simulink model "PID_discreto_vs_continuo(1)"  (R2022b)
settings: Solver=VariableStepAuto  StartTime=0.0  StopTime=5  RelTol=1e-3
undefined symbols (not defined in the file or in its folder): DiscIntNeverNeededParam
libraries: cstblocks x2, simulink x1
settings Model: Creator=57317  LastModifiedBy=Duván Ramírez Lotta

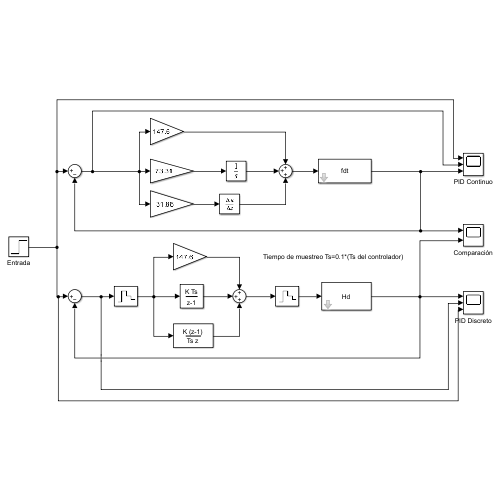
[thumbnail: Simulink's stored preview of the top-level diagram]
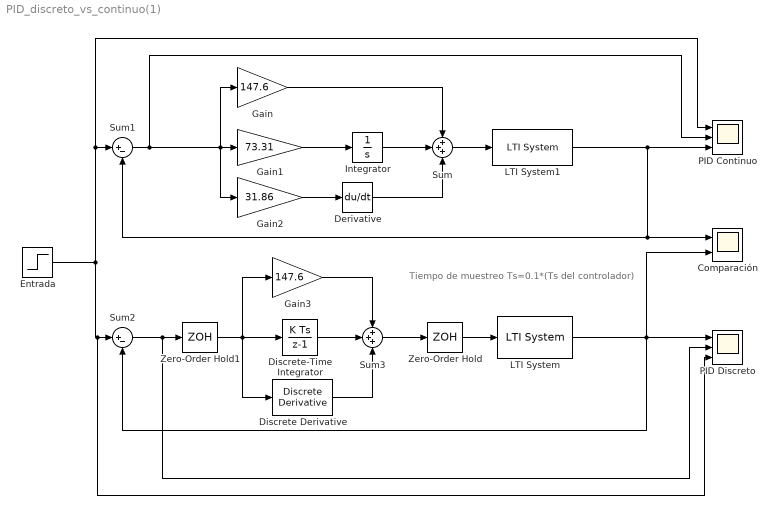
== system PID_discreto_vs_continuo(1) ==
  note: Tiempo de muestreo Ts=0.1*(Ts del controlador)
  Comparación : Scope  NumInputPorts=2
  Derivative : Derivative
  Discrete Derivative : simulink/Discrete/Discrete Derivative  gainval=31.86  ICPrevScaledInput=0.0  OutMin=[]  OutMax=[]  OutDataType=fixdt(1, 16)  OutScaling=2^-10  DoSatur=off
  Discrete-Time Integrator : DiscreteIntegrator  gainval=73.31  SampleTime=0.0001  ICPrevOutput=DiscIntNeverNeededParam  ICPrevScaledInput=DiscIntNeverNeededParam
  Entrada : Step  SampleTime=0
  Gain : Gain  Gain=147.6
  Gain1 : Gain  Gain=73.31
  Gain2 : Gain  Gain=31.86
  Gain3 : Gain  Gain=147.6
  Integrator : Integrator
  LTI System : cstblocks/LTI System  sys=Hd  IC=[]
  LTI System1 : cstblocks/LTI System  sys=fdt  IC=[]
  PID Continuo : Scope  NumInputPorts=3
  PID Discreto : Scope  NumInputPorts=3
  Sum : Sum  Inputs=+++
  Sum1 : Sum  Inputs=|+-
  Sum2 : Sum  Inputs=|+-
  Sum3 : Sum  Inputs=+++
  Zero-Order Hold : ZeroOrderHold  SampleTime=0.0001
  Zero-Order Hold1 : ZeroOrderHold  SampleTime=0.0001
  wires:
  LTI System1/1 -> PID Continuo/3, Sum1/2, Comparación/1
  Gain1/1 -> Integrator/1
  Gain/1 -> Sum/1
  Gain2/1 -> Derivative/1
  Derivative/1 -> Sum/3
  Integrator/1 -> Sum/2
  Entrada/1 -> Sum1/1, PID Continuo/1, PID Discreto/3, Sum2/1
  Sum1/1 -> PID Continuo/2, Gain/1, Gain2/1, Gain1/1
  Sum/1 -> LTI System1/1
  LTI System/1 -> Sum2/2, PID Discreto/1, Comparación/2
  Discrete-Time Integrator/1 -> Sum3/2
  Gain3/1 -> Sum3/1
  Discrete Derivative/1 -> Sum3/3
  Sum2/1 -> Zero-Order Hold1/1, PID Discreto/2
  Sum3/1 -> Zero-Order Hold/1
  Zero-Order Hold/1 -> LTI System/1
  Zero-Order Hold1/1 -> Discrete-Time Integrator/1, Gain3/1, Discrete Derivative/1
